simulink model "ARC_DTm"  (R2025b)
settings: Solver=FixedStepAuto  StartTime=0.0  StopTime=10080  FixedStep=1  RelTol=1e-3
PreLoadFcn:
  | %For Preload, set the working path
  | modelFolder = fileparts(which(bdroot));
  | addpath(genpath(modelFolder));
StartFcn:
  | tic
StopFcn:
  | fprintf("Sim Time: %.02f min", toc/60)
values from neighbouring files (symbols this model uses):
  batteryScenario = p.batteryScenario    [RUNSIM_ParameterSweep.m]    (also in _RUNSIM_ParameterSweep.m)
  Electricity_SalePriceModifier = 50/100    (= 0.5)    [RUNSIM_ParameterSweep.m]    (also in _RUNSIM_ParameterSweep.m)
  LUT = LUT_load.gamLUT    [RUNSIM_ParameterSweep.m]    (also in _RUNSIM_ParameterSweep.m)
  minimum_UF_system_flow = 5833    [RUNSIM_ParameterSweep.m]    (also in _RUNSIM_ParameterSweep.m)
  PROS1_recoveryrate = 61    [RUNSIM_ParameterSweep.m]    (also in _RUNSIM_ParameterSweep.m)
  PROS2_recoveryrate = 62    [RUNSIM_ParameterSweep.m]    (also in _RUNSIM_ParameterSweep.m)
  ROstabilization_time = p.ROstabilization_time    [RUNSIM_ParameterSweep.m]    (also in _RUNSIM_ParameterSweep.m)
  solarModifier = maximum_solar_generation / 300    [RUNSIM_ParameterSweep.m]    (also in _RUNSIM_ParameterSweep.m)
  TSRO_recoveryrate = 51    [RUNSIM_ParameterSweep.m]    (also in _RUNSIM_ParameterSweep.m)
  UF_RecoveryRate = 96    [RUNSIM_ParameterSweep.m]    (also in _RUNSIM_ParameterSweep.m)
undefined symbols (not defined in the file or in its folder): A_PROS1, A_PROS2, A_TSRO, B_PROS1, B_PROS2, B_TSRO, BW_Max_Time, BW_Max_Vol_gal, CEB_Max_Time, CEB_Max_Vol_gal, CIP_Max_Time, E, FF, h, L, w
libraries: simulink x40
(part 7 of 11)

== system ARC_DTm/Product Water Tank/Temperature Balance ==
  InflowLoadingRate1 : Inport
  InflowLoadingRate2 : Inport  Port=2
  OutflowRate1 (flow) : Inport  Port=3
  OutflowRate2 (FLOW) : Inport  Port=4
  Volume : Inport  Port=5
  *C*min^-1*VOL^-1 : Product  Inputs=*/
  *C/VOL : Integrator  InitialCondition=initT
  Outflow Rate (FLOW) : Sum  Inputs=|++
  Temperature Inflow Rate (*C/min) : Sum  Inputs=|++
  Temperature Outflow Rate (*C/m) : Product
  Total Loading Rate (*C/m) : Sum  Inputs=|+-
  Out1 : Outport
  wires:
  InflowLoadingRate1/1 -> Temperature Inflow Rate (*C/min)/1
  InflowLoadingRate2/1 -> Temperature Inflow Rate (*C/min)/2
  Temperature Inflow Rate (*C/min)/1 -> Total Loading Rate (*C/m)/1
  Total Loading Rate (*C/m)/1 -> *C*min^-1*VOL^-1/1
  Volume/1 -> *C*min^-1*VOL^-1/2
  *C*min^-1*VOL^-1/1 -> *C/VOL/1
  *C/VOL/1 -> Temperature Outflow Rate (*C/m)/1, Out1/1
  OutflowRate1 (flow)/1 -> Outflow Rate (FLOW)/1
  OutflowRate2 (FLOW)/1 -> Outflow Rate (FLOW)/2
  Outflow Rate (FLOW)/1 -> Temperature Outflow Rate (*C/m)/2
  Temperature Outflow Rate (*C/m)/1 -> Total Loading Rate (*C/m)/2

== system ARC_DTm/TSRO_1/Subsystem ==
  <Feed Temperature (oC)> : Inport
  <S2 Feed Pressure (bar)> : Inport  Port=2
  Pperm : Inport  Port=3
  Water Perm (L/m2/min/Bar) : Inport  Port=4
  Salt Perm (L/m2/min) : Inport  Port=5
  <S2 Feed Salinity (g/L)> : Inport  Port=6
  cperm : Inport  Port=7
  Jw : Inport  Port=8
  dh : Inport  Port=9
  L : Inport  Port=10
  u : Inport  Port=11
  MATLAB Function : MATLAB Function  TreatAsAtomicUnit=on
  Scope : Scope  NumInputPorts=3
      settings: ActiveDisplayYMinimum=-3.36183032878838E+280  ActiveDisplayYMaximum=3.0256472959095429E+281  DataLoggingVariableName=ScopeData26
  Scope1 : Scope
      settings: ActiveDisplayYMinimum=-1  ActiveDisplayYMaximum=1  DataLoggingVariableName=ScopeData28
  Permeate Flux Rate (L/min/m2) : Outport
  Permeate Salinity g/L : Outport  Port=2
  deltaPi_bar : Outport  Port=3
  wires:
  Salt Perm (L/m2/min)/1 -> MATLAB Function/5(B)
  <Feed Temperature (oC)>/1 -> MATLAB Function/1(T)
  <S2 Feed Salinity (g/L)>/1 -> Scope/1, MATLAB Function/6(cfeed)  "Feed Salinity g/L"
  <S2 Feed Pressure (bar)>/1 -> MATLAB Function/2(Pfeed)
  cperm/1 -> MATLAB Function/7(cperm_prev)
  Pperm/1 -> MATLAB Function/3(Pperm)
  Jw/1 -> MATLAB Function/8(Jw_prev)  "Permeate Flux (Jw)"
  Water Perm (L/m2/min/Bar)/1 -> MATLAB Function/4(A)
  dh/1 -> MATLAB Function/9(dh)
  L/1 -> MATLAB Function/10(L)
  u/1 -> MATLAB Function/11(u)  "Flow Velocity (cm/s)"
  MATLAB Function/1(Jw) -> Scope1/1, Permeate Flux Rate (L/min/m2)/1  "Permeate Flux Rate (L/min/m2)"
  MATLAB Function/2(cperm) -> Scope/2, Permeate Salinity g/L/1  "TSRO_1_PermeateSalinity_gL"
  MATLAB Function/3(deltaPi_bar) -> Scope/3, deltaPi_bar/1  "deltaPi_bar"

== system ARC_DTm/TSRO_2/Subsystem ==
  <Feed Temperature (oC)> : Inport
  <S2 Feed Pressure (bar)> : Inport  Port=2
  Pperm : Inport  Port=3
  Water Perm (L/m2/min/Bar) : Inport  Port=4
  Salt Perm (L/m2/min) : Inport  Port=5
  <S2 Feed Salinity (g/L)> : Inport  Port=6
  cperm : Inport  Port=7
  Jw : Inport  Port=8
  dh : Inport  Port=9
  L : Inport  Port=10
  u : Inport  Port=11
  MATLAB Function : MATLAB Function  TreatAsAtomicUnit=on
  Permeate Flux Rate (L/min/m2) : Outport
  Permeate Salinity g/L : Outport  Port=2
  deltaPi_bar : Outport  Port=3
  wires:
  Salt Perm (L/m2/min)/1 -> MATLAB Function/5(B)
  <Feed Temperature (oC)>/1 -> MATLAB Function/1(T)
  <S2 Feed Salinity (g/L)>/1 -> MATLAB Function/6(cfeed)  "Feed Salinity g/L"
  <S2 Feed Pressure (bar)>/1 -> MATLAB Function/2(Pfeed)
  cperm/1 -> MATLAB Function/7(cperm_prev)
  Pperm/1 -> MATLAB Function/3(Pperm)
  Jw/1 -> MATLAB Function/8(Jw_prev)  "Permeate Flux (Jw)"
  Water Perm (L/m2/min/Bar)/1 -> MATLAB Function/4(A)
  dh/1 -> MATLAB Function/9(dh)
  L/1 -> MATLAB Function/10(L)
  u/1 -> MATLAB Function/11(u)  "Flow Velocity (cm/s)"
  MATLAB Function/1(Jw) -> Permeate Flux Rate (L/min/m2)/1  "Permeate Flux Rate (L/min/m2)"
  MATLAB Function/2(cperm) -> Permeate Salinity g/L/1  "TSRO_2_PermeateSalinity_gL"
  MATLAB Function/3(deltaPi_bar) -> deltaPi_bar/1

== system ARC_DTm/TSRO_3/Subsystem ==
  <Feed Temperature (oC)> : Inport
  <S2 Feed Pressure (bar)> : Inport  Port=2
  Pperm : Inport  Port=3
  Water Perm (L/m2/min/Bar) : Inport  Port=4
  Salt Perm (L/m2/min) : Inport  Port=5
  <S2 Feed Salinity (g/L)> : Inport  Port=6
  cperm : Inport  Port=7
  Jw : Inport  Port=8
  dh : Inport  Port=9
  L : Inport  Port=10
  u : Inport  Port=11
  MATLAB Function : MATLAB Function  TreatAsAtomicUnit=on
  Permeate Flux Rate (L/min/m2) : Outport
  Permeate Salinity g/L : Outport  Port=2
  deltaPi_bar : Outport  Port=3
  wires:
  Salt Perm (L/m2/min)/1 -> MATLAB Function/5(B)
  <Feed Temperature (oC)>/1 -> MATLAB Function/1(T)
  <S2 Feed Salinity (g/L)>/1 -> MATLAB Function/6(cfeed)  "Feed Salinity g/L"
  <S2 Feed Pressure (bar)>/1 -> MATLAB Function/2(Pfeed)
  cperm/1 -> MATLAB Function/7(cperm_prev)
  Pperm/1 -> MATLAB Function/3(Pperm)
  Jw/1 -> MATLAB Function/8(Jw_prev)  "Permeate Flux (Jw)"
  Water Perm (L/m2/min/Bar)/1 -> MATLAB Function/4(A)
  dh/1 -> MATLAB Function/9(dh)
  L/1 -> MATLAB Function/10(L)
  u/1 -> MATLAB Function/11(u)  "Flow Velocity (cm/s)"
  MATLAB Function/1(Jw) -> Permeate Flux Rate (L/min/m2)/1  "Permeate Flux Rate (L/min/m2)"
  MATLAB Function/2(cperm) -> Permeate Salinity g/L/1  "TSRO_3_PermeateSalinity_gL"
  MATLAB Function/3(deltaPi_bar) -> deltaPi_bar/1

== system ARC_DTm/TSRO_4/Subsystem ==
  <Feed Temperature (oC)> : Inport
  <S2 Feed Pressure (bar)> : Inport  Port=2
  Pperm : Inport  Port=3
  Water Perm (L/m2/min/Bar) : Inport  Port=4
  Salt Perm (L/m2/min) : Inport  Port=5
  <S2 Feed Salinity (g/L)> : Inport  Port=6
  cperm : Inport  Port=7
  Jw : Inport  Port=8
  dh : Inport  Port=9
  L : Inport  Port=10
  u : Inport  Port=11
  MATLAB Function : MATLAB Function  TreatAsAtomicUnit=on
  Permeate Flux Rate (L/min/m2) : Outport
  Permeate Salinity g/L : Outport  Port=2
  deltaPi_bar : Outport  Port=3
  wires:
  Salt Perm (L/m2/min)/1 -> MATLAB Function/5(B)
  <Feed Temperature (oC)>/1 -> MATLAB Function/1(T)
  <S2 Feed Salinity (g/L)>/1 -> MATLAB Function/6(cfeed)  "Feed Salinity g/L"
  <S2 Feed Pressure (bar)>/1 -> MATLAB Function/2(Pfeed)
  cperm/1 -> MATLAB Function/7(cperm_prev)
  Pperm/1 -> MATLAB Function/3(Pperm)
  Jw/1 -> MATLAB Function/8(Jw_prev)  "Permeate Flux (Jw)"
  Water Perm (L/m2/min/Bar)/1 -> MATLAB Function/4(A)
  dh/1 -> MATLAB Function/9(dh)
  L/1 -> MATLAB Function/10(L)
  u/1 -> MATLAB Function/11(u)  "Flow Velocity (cm/s)"
  MATLAB Function/1(Jw) -> Permeate Flux Rate (L/min/m2)/1  "Permeate Flux Rate (L/min/m2)"
  MATLAB Function/2(cperm) -> Permeate Salinity g/L/1  "TSRO_4_PermeateSalinity_gL"
  MATLAB Function/3(deltaPi_bar) -> deltaPi_bar/1

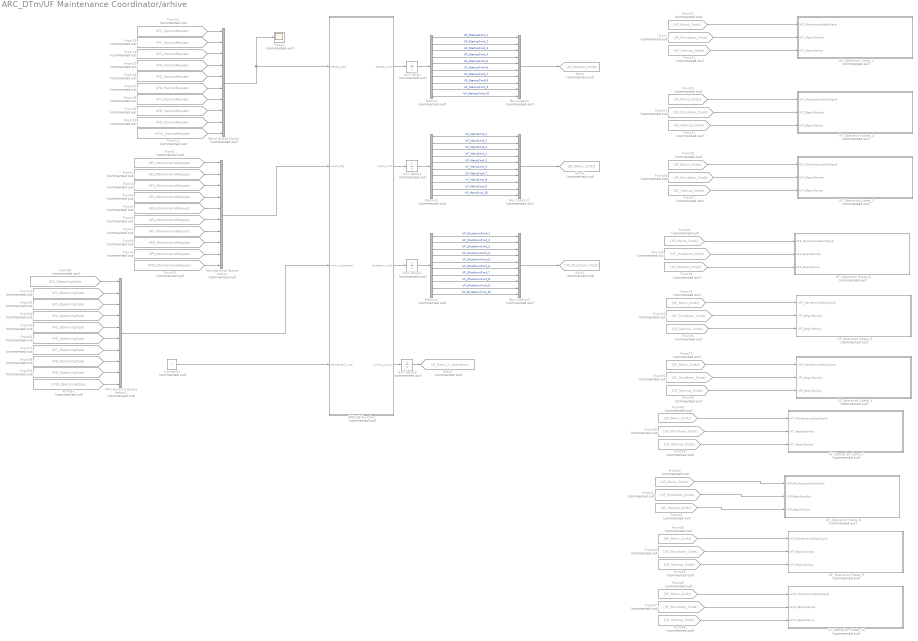
== system ARC_DTm/UF Maintenance Coordinator/arhive ==
  Bus Creator : BusCreator  Commented=on  Inputs=10
  Bus Creator1 : BusCreator  Commented=on  Inputs=10
  Bus Creator2 : BusCreator  Commented=on  Inputs=10
  Constant1 : Constant  Commented=on  Value=7
  Demux : Demux  Commented=on  Outputs=10
  Demux1 : Demux  Commented=on  Outputs=10
  Demux2 : Demux  Commented=on  Outputs=10
  From{,23,26,29,32,35,38,41,44,47} (10 alike) : From  Commented=on  GotoTag=UF_Shutdown_Cmds
  From1 : From  Commented=on  GotoTag=UF1_MaintenanceRequest  TagVisibility=global
  From10 : From  Commented=on  GotoTag=UF10_MaintenanceRequest  TagVisibility=global
  From11 : From  Commented=on  GotoTag=UF1_StartupRequest  TagVisibility=global
  From12 : From  Commented=on  GotoTag=UF10_StartupRequest  TagVisibility=global
  From13 : From  Commented=on  GotoTag=UF2_StartupRequest  TagVisibility=global
  From14 : From  Commented=on  GotoTag=UF3_StartupRequest  TagVisibility=global
  From15 : From  Commented=on  GotoTag=UF4_StartupRequest  TagVisibility=global
  From16 : From  Commented=on  GotoTag=UF5_StartupRequest  TagVisibility=global
  From17 : From  Commented=on  GotoTag=UF6_StartupRequest  TagVisibility=global
  From18 : From  Commented=on  GotoTag=UF7_StartupRequest  TagVisibility=global
  From19 : From  Commented=on  GotoTag=UF8_StartupRequest  TagVisibility=global
  From2 : From  Commented=on  GotoTag=UF2_MaintenanceRequest  TagVisibility=global
  From20 : From  Commented=on  GotoTag=UF9_StartupRequest  TagVisibility=global
  From{21,24,27,30,33,36,39,42,45,48} (10 alike) : From  Commented=on  GotoTag=UF_Startup_Cmds
  From{22,25,28,31,34,37,40,43,46,49} (10 alike) : From  Commented=on  GotoTag=UF_Maint_Cmds
  From3 : From  Commented=on  GotoTag=UF3_MaintenanceRequest  TagVisibility=global
  From4 : From  Commented=on  GotoTag=UF4_MaintenanceRequest  TagVisibility=global
  From5 : From  Commented=on  GotoTag=UF5_MaintenanceRequest  TagVisibility=global
  From50 : From  Commented=on  GotoTag=UF1_OperatingState  TagVisibility=global
  From51 : From  Commented=on  GotoTag=UF10_OperatingState  TagVisibility=global
  From52 : From  Commented=on  GotoTag=UF2_OperatingState  TagVisibility=global
  From53 : From  Commented=on  GotoTag=UF3_OperatingState  TagVisibility=global
  From54 : From  Commented=on  GotoTag=UF4_OperatingState  TagVisibility=global
  From55 : From  Commented=on  GotoTag=UF5_OperatingState  TagVisibility=global
  From56 : From  Commented=on  GotoTag=UF6_OperatingState  TagVisibility=global
  From57 : From  Commented=on  GotoTag=UF7_OperatingState  TagVisibility=global
  From58 : From  Commented=on  GotoTag=UF8_OperatingState  TagVisibility=global
  From59 : From  Commented=on  GotoTag=UF9_OperatingState  TagVisibility=global
  From6 : From  Commented=on  GotoTag=UF6_MaintenanceRequest  TagVisibility=global
  From7 : From  Commented=on  GotoTag=UF7_MaintenanceRequest  TagVisibility=global
  From8 : From  Commented=on  GotoTag=UF8_MaintenanceRequest  TagVisibility=global
  From9 : From  Commented=on  GotoTag=UF9_MaintenanceRequest  TagVisibility=global
  Goto : Goto  Commented=on  GotoTag=UF_Startup_Cmds
  Goto1 : Goto  Commented=on  GotoTag=UF_Maint_Cmds
  Goto2 : Goto  Commented=on  GotoTag=UF_Shutdown_Cmds
  Goto3 : Goto  Commented=on  GotoTag=UF_Units_in_operations  TagVisibility=global
  MATLAB Function : MATLAB Function  Priority=100  Commented=on  TreatAsAtomicUnit=on
  Maint Queue Vector : Mux  Commented=on  Inputs=10
  Maintenance Queue Vector : Mux  Commented=on  Inputs=10
  Maintenance Queue Vector1 : Mux  Commented=on  Inputs=10
  Scope : Scope  Commented=on
      settings: ActiveDisplayYMinimum=0.31827009128781919  ActiveDisplayYMaximum=0.91954146390153213
  UF_Operation State_1 : Subsystem  Commented=on
  UF_Operation State_10 : Subsystem  Commented=on
  UF_Operation State_2 : Subsystem  Commented=on
  UF_Operation State_3 : Subsystem  Commented=on
  UF_Operation State_4 : Subsystem  Commented=on
  UF_Operation State_5 : Subsystem  Commented=on
  UF_Operation State_6 : Subsystem  Commented=on
  UF_Operation State_7 : Subsystem  Commented=on
  UF_Operation State_8 : Subsystem  Commented=on
  UF_Operation State_9 : Subsystem  Commented=on
  Unit Delay{,1..3} (4 alike) : UnitDelay  Commented=on  SampleTime=-1  HasFrameUpgradeWarning=on
  wires:
  Demux2/9 -> Bus Creator2/9  "UF_ShutdownCmd_9"
  From13/1 -> Maint Queue Vector/2
  From42/1 -> UF_Operation State_8/3(UF8_BeginStartup)
  From48/1 -> UF_Operation State_10/3(UF10_BeginStartup)
  Demux2/10 -> Bus Creator2/10  "UF_ShutdownCmd_10"
  From47/1 -> UF_Operation State_10/2(UF10_BeginStandby)
  Demux2/6 -> Bus Creator2/6  "UF_ShutdownCmd_6"
  Demux1/6 -> Bus Creator1/6  "UF_MaintCmd_6"
  From24/1 -> UF_Operation State_2/3(UF2_BeginStartup)
  Maintenance Queue Vector/1 -> MATLAB Function/2(maint_req)
  From1/1 -> Maintenance Queue Vector/1
  From23/1 -> UF_Operation State_2/2(UF2_BeginStandby)
  MATLAB Function/3(shutdown_cmd) -> Unit Delay2/1
  From30/1 -> UF_Operation State_4/3(UF4_BeginStartup)
  From57/1 -> Maintenance Queue Vector1/7
  Unit Delay/1 -> Demux/1
  Demux/10 -> Bus Creator/10  "UF_StartupCmd_10"
  From54/1 -> Maintenance Queue Vector1/4
  From45/1 -> UF_Operation State_9/3(UF9_BeginStartup)
  Demux1/2 -> Bus Creator1/2  "UF_MaintCmd_2"
  From7/1 -> Maintenance Queue Vector/7
  From58/1 -> Maintenance Queue Vector1/8
  From49/1 -> UF_Operation State_10/1(UF10_MaintenanceStartSignal)
  From29/1 -> UF_Operation State_4/2(UF4_BeginStandby)
  From6/1 -> Maintenance Queue Vector/6
  From10/1 -> Maintenance Queue Vector/10
  From56/1 -> Maintenance Queue Vector1/6
  From33/1 -> UF_Operation State_5/3(UF5_BeginStartup)
  From31/1 -> UF_Operation State_4/1(UF4_MaintenanceStartSignal)
  From/1 -> UF_Operation State_1/2(UF1_BeginStandby)
  From53/1 -> Maintenance Queue Vector1/3
  From34/1 -> UF_Operation State_5/1(UF5_MaintenanceStartSignal)
  Demux2/5 -> Bus Creator2/5  "UF_ShutdownCmd_5"
  Unit Delay3/1 -> Goto3/1
  From59/1 -> Maintenance Queue Vector1/9
  Demux/7 -> Bus Creator/7  "UF_StartupCmd_7"
  Maintenance Queue Vector1/1 -> MATLAB Function/3(unit_in_operation)
  Demux2/7 -> Bus Creator2/7  "UF_ShutdownCmd_7"
  From3/1 -> Maintenance Queue Vector/3
  From38/1 -> UF_Operation State_7/2(UF7_BeginStandby)
  From40/1 -> UF_Operation State_7/1(UF7_MaintenanceStartSignal)
  From26/1 -> UF_Operation State_3/2(UF3_BeginStandby)
  Bus Creator1/1 -> Goto1/1
  From2/1 -> Maintenance Queue Vector/2
  Demux2/3 -> Bus Creator2/3  "UF_ShutdownCmd_3"
  From39/1 -> UF_Operation State_7/3(UF7_BeginStartup)
  Demux1/9 -> Bus Creator1/9  "UF_MaintCmd_9"
  Demux2/2 -> Bus Creator2/2  "UF_ShutdownCmd_2"
  From46/1 -> UF_Operation State_9/1(UF9_MaintenanceStartSignal)
  From20/1 -> Maint Queue Vector/9
  Demux/4 -> Bus Creator/4  "UF_StartupCmd_4"
  Demux2/4 -> Bus Creator2/4  "UF_ShutdownCmd_4"
  Demux/5 -> Bus Creator/5  "UF_StartupCmd_5"
  Demux2/1 -> Bus Creator2/1  "UF_ShutdownCmd_1"
  From9/1 -> Maintenance Queue Vector/9
  From32/1 -> UF_Operation State_5/2(UF5_BeginStandby)
  Demux1/3 -> Bus Creator1/3  "UF_MaintCmd_3"
  Demux1/5 -> Bus Creator1/5  "UF_MaintCmd_5"
  From55/1 -> Maintenance Queue Vector1/5
  From4/1 -> Maintenance Queue Vector/4
  MATLAB Function/4(running_count) -> Unit Delay3/1
  Demux/6 -> Bus Creator/6  "UF_StartupCmd_6"
  From22/1 -> UF_Operation State_1/1(UF1_MaintenanceStartSignal)
  Demux/8 -> Bus Creator/8  "UF_StartupCmd_8"
  Demux/9 -> Bus Creator/9  "UF_StartupCmd_9"
  From8/1 -> Maintenance Queue Vector/8
  Demux1/1 -> Bus Creator1/1  "UF_MaintCmd_1"
  Demux1/10 -> Bus Creator1/10  "UF_MaintCmd_10"
  From50/1 -> Maintenance Queue Vector1/1
  Demux1/4 -> Bus Creator1/4  "UF_MaintCmd_4"
  MATLAB Function/1(startup_cmd) -> Unit Delay/1
  From52/1 -> Maintenance Queue Vector1/2
  From27/1 -> UF_Operation State_3/3(UF3_BeginStartup)
  From15/1 -> Maint Queue Vector/4
  From51/1 -> Maintenance Queue Vector1/10
  From36/1 -> UF_Operation State_6/3(UF6_BeginStartup)
  MATLAB Function/2(maint_cmd) -> Unit Delay1/1
  Unit Delay2/1 -> Demux2/1
  From43/1 -> UF_Operation State_8/1(UF8_MaintenanceStartSignal)
  From28/1 -> UF_Operation State_3/1(UF3_MaintenanceStartSignal)
  Demux2/8 -> Bus Creator2/8  "UF_ShutdownCmd_8"
  Demux/2 -> Bus Creator/2  "UF_StartupCmd_2"
  From35/1 -> UF_Operation State_6/2(UF6_BeginStandby)
  Bus Creator2/1 -> Goto2/1
  Bus Creator/1 -> Goto/1
  From37/1 -> UF_Operation State_6/1(UF6_MaintenanceStartSignal)
  Constant1/1 -> MATLAB Function/4(demanded_units)
  Demux1/8 -> Bus Creator1/8  "UF_MaintCmd_8"
  From25/1 -> UF_Operation State_2/1(UF2_MaintenanceStartSignal)
  From44/1 -> UF_Operation State_9/2(UF9_BeginStandby)
  Demux1/7 -> Bus Creator1/7  "UF_MaintCmd_7"
  Demux/3 -> Bus Creator/3  "UF_StartupCmd_3"
  Demux/1 -> Bus Creator/1  "UF_StartupCmd_1"
  From41/1 -> UF_Operation State_8/2(UF8_BeginStandby)
  From21/1 -> UF_Operation State_1/3(UF1_BeginStartup)
  From5/1 -> Maintenance Queue Vector/5
  Unit Delay1/1 -> Demux1/1
  From16/1 -> Maint Queue Vector/5
  From17/1 -> Maint Queue Vector/6
  From19/1 -> Maint Queue Vector/8
  From11/1 -> Maint Queue Vector/1
  From12/1 -> Maint Queue Vector/10
  From18/1 -> Maint Queue Vector/7
  Maint Queue Vector/1 -> Scope/1, MATLAB Function/1(startup_req)
  From14/1 -> Maint Queue Vector/3

== system ARC_DTm/UF1/Subsystem ==
  note: The GAM utilizes smoothing functions to generate non-interacting linear regressions between the parameters. The format of the equation is as such:
      | $y = \beta_0 + \sum_{n=1}^N{f_n(x_n)}\\ f_n(x_n) = \beta_{n}*sm_n(x_n)$
      | where f_n is the weighted smoothing function for variable n across the set N. Each 1-D lookup table below represents the weighted smooth function output for the respective variable. This GAM lookup table approach provided a more computationally efficient method to predict using the GAM at very minor losses in fidelity ( ~0.1% MAPE from raw GAM outputs across a test set).
  t_BW : Inport
  t_CEB : Inport  Port=2
  t_CIP : Inport  Port=3
  V_BW : Inport  Port=4
  V_CEB : Inport  Port=5
  Feed Turbidity : Inport  Port=6
  T : Inport  Port=7
  B1: t_BW : Lookup_n-D  NumberOfTableDimensions=1  BreakpointsForDimension1=LUT.breakpoints(:,3)  Table=LUT.values(:,3)  ExtrapMethod=Clip  InternalRulePriority=Speed  RndMeth=Simplest
  B2: t_CEB : Lookup_n-D  NumberOfTableDimensions=1  BreakpointsForDimension1=LUT.breakpoints(:,5)  Table=LUT.values(:,5)  ExtrapMethod=Clip  InternalRulePriority=Speed  RndMeth=Simplest
  B3: t_CIP : Lookup_n-D  NumberOfTableDimensions=1  BreakpointsForDimension1=LUT.breakpoints(:,4)  Table=LUT.values(:,4)  ExtrapMethod=Clip  InternalRulePriority=Speed  RndMeth=Simplest
  B4: V_BW : Lookup_n-D  NumberOfTableDimensions=1  BreakpointsForDimension1=LUT.breakpoints(:,6)  Table=LUT.values(:,6)  ExtrapMethod=Clip  InternalRulePriority=Speed  RndMeth=Simplest
  B5: V_CEB : Lookup_n-D  NumberOfTableDimensions=1  BreakpointsForDimension1=LUT.breakpoints(:,7)  Table=LUT.values(:,7)  ExtrapMethod=Clip  InternalRulePriority=Speed  RndMeth=Simplest
  B6: Turbidity : Lookup_n-D  NumberOfTableDimensions=1  BreakpointsForDimension1=LUT.breakpoints(:,1)  Table=LUT.values(:,1)  ExtrapMethod=Clip  InternalRulePriority=Speed  RndMeth=Simplest
  B7: Temperature : Lookup_n-D  NumberOfTableDimensions=1  BreakpointsForDimension1=LUT.breakpoints(:,2)  Table=LUT.values(:,2)  ExtrapMethod=Clip  InternalRulePriority=Speed  RndMeth=Simplest
  Intercept : Constant  Value=LUT.intercept
  Sum : Sum  Inputs=++++++++
  A_UF : Outport
  wires:
  Sum/1 -> A_UF/1
  t_BW/1 -> B1: t_BW/1
  B1: t_BW/1 -> Sum/2
  Intercept/1 -> Sum/1
  t_CEB/1 -> B2: t_CEB/1
  B2: t_CEB/1 -> Sum/3
  t_CIP/1 -> B3: t_CIP/1
  B3: t_CIP/1 -> Sum/4
  V_BW/1 -> B4: V_BW/1
  B4: V_BW/1 -> Sum/5
  V_CEB/1 -> B5: V_CEB/1
  B5: V_CEB/1 -> Sum/6
  B6: Turbidity/1 -> Sum/7
  Feed Turbidity/1 -> B6: Turbidity/1
  T/1 -> B7: Temperature/1
  B7: Temperature/1 -> Sum/8

== system ARC_DTm/UF10/Subsystem ==
  note: The GAM utilizes smoothing functions to generate non-interacting linear regressions between the parameters. The format of the equation is as such:
      | $y = \beta_0 + \sum_{n=1}^N{f_n(x_n)}\\ f_n(x_n) = \beta_{n}*sm_n(x_n)$
      | where f_n is the weighted smoothing function for variable n across the set N. Each 1-D lookup table below represents the weighted smooth function output for the respective variable. This GAM lookup table approach provided a more computationally efficient method to predict using the GAM at very minor losses in fidelity ( ~0.1% MAPE from raw GAM outputs across a test set).
  t_BW : Inport
  t_CEB : Inport  Port=2
  t_CIP : Inport  Port=3
  V_BW : Inport  Port=4
  V_CEB : Inport  Port=5
  Feed Turbidity : Inport  Port=6
  T : Inport  Port=7
  B1: t_BW : Lookup_n-D  NumberOfTableDimensions=1  BreakpointsForDimension1=LUT.breakpoints(:,3)  Table=LUT.values(:,3)  ExtrapMethod=Clip  InternalRulePriority=Speed  RndMeth=Simplest
  B2: t_CEB : Lookup_n-D  NumberOfTableDimensions=1  BreakpointsForDimension1=LUT.breakpoints(:,5)  Table=LUT.values(:,5)  ExtrapMethod=Clip  InternalRulePriority=Speed  RndMeth=Simplest
  B3: t_CIP : Lookup_n-D  NumberOfTableDimensions=1  BreakpointsForDimension1=LUT.breakpoints(:,4)  Table=LUT.values(:,4)  ExtrapMethod=Clip  InternalRulePriority=Speed  RndMeth=Simplest
  B4: V_BW : Lookup_n-D  NumberOfTableDimensions=1  BreakpointsForDimension1=LUT.breakpoints(:,6)  Table=LUT.values(:,6)  ExtrapMethod=Clip  InternalRulePriority=Speed  RndMeth=Simplest
  B5: V_CEB : Lookup_n-D  NumberOfTableDimensions=1  BreakpointsForDimension1=LUT.breakpoints(:,7)  Table=LUT.values(:,7)  ExtrapMethod=Clip  InternalRulePriority=Speed  RndMeth=Simplest
  B6: Turbidity : Lookup_n-D  NumberOfTableDimensions=1  BreakpointsForDimension1=LUT.breakpoints(:,1)  Table=LUT.values(:,1)  ExtrapMethod=Clip  InternalRulePriority=Speed  RndMeth=Simplest
  B7: Temperature : Lookup_n-D  NumberOfTableDimensions=1  BreakpointsForDimension1=LUT.breakpoints(:,2)  Table=LUT.values(:,2)  ExtrapMethod=Clip  InternalRulePriority=Speed  RndMeth=Simplest
  Intercept : Constant  Value=LUT.intercept
  Sum : Sum  Inputs=++++++++
  A_UF : Outport
  wires:
  Sum/1 -> A_UF/1
  t_BW/1 -> B1: t_BW/1
  B1: t_BW/1 -> Sum/2
  Intercept/1 -> Sum/1
  t_CEB/1 -> B2: t_CEB/1
  B2: t_CEB/1 -> Sum/3
  t_CIP/1 -> B3: t_CIP/1
  B3: t_CIP/1 -> Sum/4
  V_BW/1 -> B4: V_BW/1
  B4: V_BW/1 -> Sum/5
  V_CEB/1 -> B5: V_CEB/1
  B5: V_CEB/1 -> Sum/6
  B6: Turbidity/1 -> Sum/7
  Feed Turbidity/1 -> B6: Turbidity/1
  T/1 -> B7: Temperature/1
  B7: Temperature/1 -> Sum/8

== system ARC_DTm/UF2/Subsystem ==
  note: The GAM utilizes smoothing functions to generate non-interacting linear regressions between the parameters. The format of the equation is as such:
      | $y = \beta_0 + \sum_{n=1}^N{f_n(x_n)}\\ f_n(x_n) = \beta_{n}*sm_n(x_n)$
      | where f_n is the weighted smoothing function for variable n across the set N. Each 1-D lookup table below represents the weighted smooth function output for the respective variable. This GAM lookup table approach provided a more computationally efficient method to predict using the GAM at very minor losses in fidelity ( ~0.1% MAPE from raw GAM outputs across a test set).
  t_BW : Inport
  t_CEB : Inport  Port=2
  t_CIP : Inport  Port=3
  V_BW : Inport  Port=4
  V_CEB : Inport  Port=5
  Feed Turbidity : Inport  Port=6
  T : Inport  Port=7
  B1: t_BW : Lookup_n-D  NumberOfTableDimensions=1  BreakpointsForDimension1=LUT.breakpoints(:,3)  Table=LUT.values(:,3)  ExtrapMethod=Clip  InternalRulePriority=Speed  RndMeth=Simplest
  B2: t_CEB : Lookup_n-D  NumberOfTableDimensions=1  BreakpointsForDimension1=LUT.breakpoints(:,5)  Table=LUT.values(:,5)  ExtrapMethod=Clip  InternalRulePriority=Speed  RndMeth=Simplest
  B3: t_CIP : Lookup_n-D  NumberOfTableDimensions=1  BreakpointsForDimension1=LUT.breakpoints(:,4)  Table=LUT.values(:,4)  ExtrapMethod=Clip  InternalRulePriority=Speed  RndMeth=Simplest
  B4: V_BW : Lookup_n-D  NumberOfTableDimensions=1  BreakpointsForDimension1=LUT.breakpoints(:,6)  Table=LUT.values(:,6)  ExtrapMethod=Clip  InternalRulePriority=Speed  RndMeth=Simplest
  B5: V_CEB : Lookup_n-D  NumberOfTableDimensions=1  BreakpointsForDimension1=LUT.breakpoints(:,7)  Table=LUT.values(:,7)  ExtrapMethod=Clip  InternalRulePriority=Speed  RndMeth=Simplest
  B6: Turbidity : Lookup_n-D  NumberOfTableDimensions=1  BreakpointsForDimension1=LUT.breakpoints(:,1)  Table=LUT.values(:,1)  ExtrapMethod=Clip  InternalRulePriority=Speed  RndMeth=Simplest
  B7: Temperature : Lookup_n-D  NumberOfTableDimensions=1  BreakpointsForDimension1=LUT.breakpoints(:,2)  Table=LUT.values(:,2)  ExtrapMethod=Clip  InternalRulePriority=Speed  RndMeth=Simplest
  Intercept : Constant  Value=LUT.intercept
  Sum : Sum  Inputs=++++++++
  A_UF : Outport
  wires:
  Sum/1 -> A_UF/1
  t_BW/1 -> B1: t_BW/1
  B1: t_BW/1 -> Sum/2
  Intercept/1 -> Sum/1
  t_CEB/1 -> B2: t_CEB/1
  B2: t_CEB/1 -> Sum/3
  t_CIP/1 -> B3: t_CIP/1
  B3: t_CIP/1 -> Sum/4
  V_BW/1 -> B4: V_BW/1
  B4: V_BW/1 -> Sum/5
  V_CEB/1 -> B5: V_CEB/1
  B5: V_CEB/1 -> Sum/6
  B6: Turbidity/1 -> Sum/7
  Feed Turbidity/1 -> B6: Turbidity/1
  T/1 -> B7: Temperature/1
  B7: Temperature/1 -> Sum/8

== system ARC_DTm/UF3/Subsystem ==
  note: The GAM utilizes smoothing functions to generate non-interacting linear regressions between the parameters. The format of the equation is as such:
      | $y = \beta_0 + \sum_{n=1}^N{f_n(x_n)}\\ f_n(x_n) = \beta_{n}*sm_n(x_n)$
      | where f_n is the weighted smoothing function for variable n across the set N. Each 1-D lookup table below represents the weighted smooth function output for the respective variable. This GAM lookup table approach provided a more computationally efficient method to predict using the GAM at very minor losses in fidelity ( ~0.1% MAPE from raw GAM outputs across a test set).
  t_BW : Inport
  t_CEB : Inport  Port=2
  t_CIP : Inport  Port=3
  V_BW : Inport  Port=4
  V_CEB : Inport  Port=5
  Feed Turbidity : Inport  Port=6
  T : Inport  Port=7
  B1: t_BW : Lookup_n-D  NumberOfTableDimensions=1  BreakpointsForDimension1=LUT.breakpoints(:,3)  Table=LUT.values(:,3)  ExtrapMethod=Clip  InternalRulePriority=Speed  RndMeth=Simplest
  B2: t_CEB : Lookup_n-D  NumberOfTableDimensions=1  BreakpointsForDimension1=LUT.breakpoints(:,5)  Table=LUT.values(:,5)  ExtrapMethod=Clip  InternalRulePriority=Speed  RndMeth=Simplest
  B3: t_CIP : Lookup_n-D  NumberOfTableDimensions=1  BreakpointsForDimension1=LUT.breakpoints(:,4)  Table=LUT.values(:,4)  ExtrapMethod=Clip  InternalRulePriority=Speed  RndMeth=Simplest
  B4: V_BW : Lookup_n-D  NumberOfTableDimensions=1  BreakpointsForDimension1=LUT.breakpoints(:,6)  Table=LUT.values(:,6)  ExtrapMethod=Clip  InternalRulePriority=Speed  RndMeth=Simplest
  B5: V_CEB : Lookup_n-D  NumberOfTableDimensions=1  BreakpointsForDimension1=LUT.breakpoints(:,7)  Table=LUT.values(:,7)  ExtrapMethod=Clip  InternalRulePriority=Speed  RndMeth=Simplest
  B6: Turbidity : Lookup_n-D  NumberOfTableDimensions=1  BreakpointsForDimension1=LUT.breakpoints(:,1)  Table=LUT.values(:,1)  ExtrapMethod=Clip  InternalRulePriority=Speed  RndMeth=Simplest
  B7: Temperature : Lookup_n-D  NumberOfTableDimensions=1  BreakpointsForDimension1=LUT.breakpoints(:,2)  Table=LUT.values(:,2)  ExtrapMethod=Clip  InternalRulePriority=Speed  RndMeth=Simplest
  Intercept : Constant  Value=LUT.intercept
  Sum : Sum  Inputs=++++++++
  A_UF : Outport
  wires:
  Sum/1 -> A_UF/1
  t_BW/1 -> B1: t_BW/1
  B1: t_BW/1 -> Sum/2
  Intercept/1 -> Sum/1
  t_CEB/1 -> B2: t_CEB/1
  B2: t_CEB/1 -> Sum/3
  t_CIP/1 -> B3: t_CIP/1
  B3: t_CIP/1 -> Sum/4
  V_BW/1 -> B4: V_BW/1
  B4: V_BW/1 -> Sum/5
  V_CEB/1 -> B5: V_CEB/1
  B5: V_CEB/1 -> Sum/6
  B6: Turbidity/1 -> Sum/7
  Feed Turbidity/1 -> B6: Turbidity/1
  T/1 -> B7: Temperature/1
  B7: Temperature/1 -> Sum/8

== system ARC_DTm/UF4/Subsystem ==
  note: The GAM utilizes smoothing functions to generate non-interacting linear regressions between the parameters. The format of the equation is as such:
      | $y = \beta_0 + \sum_{n=1}^N{f_n(x_n)}\\ f_n(x_n) = \beta_{n}*sm_n(x_n)$
      | where f_n is the weighted smoothing function for variable n across the set N. Each 1-D lookup table below represents the weighted smooth function output for the respective variable. This GAM lookup table approach provided a more computationally efficient method to predict using the GAM at very minor losses in fidelity ( ~0.1% MAPE from raw GAM outputs across a test set).
  t_BW : Inport
  t_CEB : Inport  Port=2
  t_CIP : Inport  Port=3
  V_BW : Inport  Port=4
  V_CEB : Inport  Port=5
  Feed Turbidity : Inport  Port=6
  T : Inport  Port=7
  B1: t_BW : Lookup_n-D  NumberOfTableDimensions=1  BreakpointsForDimension1=LUT.breakpoints(:,3)  Table=LUT.values(:,3)  ExtrapMethod=Clip  InternalRulePriority=Speed  RndMeth=Simplest
  B2: t_CEB : Lookup_n-D  NumberOfTableDimensions=1  BreakpointsForDimension1=LUT.breakpoints(:,5)  Table=LUT.values(:,5)  ExtrapMethod=Clip  InternalRulePriority=Speed  RndMeth=Simplest
  B3: t_CIP : Lookup_n-D  NumberOfTableDimensions=1  BreakpointsForDimension1=LUT.breakpoints(:,4)  Table=LUT.values(:,4)  ExtrapMethod=Clip  InternalRulePriority=Speed  RndMeth=Simplest
  B4: V_BW : Lookup_n-D  NumberOfTableDimensions=1  BreakpointsForDimension1=LUT.breakpoints(:,6)  Table=LUT.values(:,6)  ExtrapMethod=Clip  InternalRulePriority=Speed  RndMeth=Simplest
  B5: V_CEB : Lookup_n-D  NumberOfTableDimensions=1  BreakpointsForDimension1=LUT.breakpoints(:,7)  Table=LUT.values(:,7)  ExtrapMethod=Clip  InternalRulePriority=Speed  RndMeth=Simplest
  B6: Turbidity : Lookup_n-D  NumberOfTableDimensions=1  BreakpointsForDimension1=LUT.breakpoints(:,1)  Table=LUT.values(:,1)  ExtrapMethod=Clip  InternalRulePriority=Speed  RndMeth=Simplest
  B7: Temperature : Lookup_n-D  NumberOfTableDimensions=1  BreakpointsForDimension1=LUT.breakpoints(:,2)  Table=LUT.values(:,2)  ExtrapMethod=Clip  InternalRulePriority=Speed  RndMeth=Simplest
  Intercept : Constant  Value=LUT.intercept
  Sum : Sum  Inputs=++++++++
  A_UF : Outport
  wires:
  Sum/1 -> A_UF/1
  t_BW/1 -> B1: t_BW/1
  B1: t_BW/1 -> Sum/2
  Intercept/1 -> Sum/1
  t_CEB/1 -> B2: t_CEB/1
  B2: t_CEB/1 -> Sum/3
  t_CIP/1 -> B3: t_CIP/1
  B3: t_CIP/1 -> Sum/4
  V_BW/1 -> B4: V_BW/1
  B4: V_BW/1 -> Sum/5
  V_CEB/1 -> B5: V_CEB/1
  B5: V_CEB/1 -> Sum/6
  B6: Turbidity/1 -> Sum/7
  Feed Turbidity/1 -> B6: Turbidity/1
  T/1 -> B7: Temperature/1
  B7: Temperature/1 -> Sum/8

== system ARC_DTm/UF5/Subsystem ==
  note: The GAM utilizes smoothing functions to generate non-interacting linear regressions between the parameters. The format of the equation is as such:
      | $y = \beta_0 + \sum_{n=1}^N{f_n(x_n)}\\ f_n(x_n) = \beta_{n}*sm_n(x_n)$
      | where f_n is the weighted smoothing function for variable n across the set N. Each 1-D lookup table below represents the weighted smooth function output for the respective variable. This GAM lookup table approach provided a more computationally efficient method to predict using the GAM at very minor losses in fidelity ( ~0.1% MAPE from raw GAM outputs across a test set).
  t_BW : Inport
  t_CEB : Inport  Port=2
  t_CIP : Inport  Port=3
  V_BW : Inport  Port=4
  V_CEB : Inport  Port=5
  Feed Turbidity : Inport  Port=6
  T : Inport  Port=7
  B1: t_BW : Lookup_n-D  NumberOfTableDimensions=1  BreakpointsForDimension1=LUT.breakpoints(:,3)  Table=LUT.values(:,3)  ExtrapMethod=Clip  InternalRulePriority=Speed  RndMeth=Simplest
  B2: t_CEB : Lookup_n-D  NumberOfTableDimensions=1  BreakpointsForDimension1=LUT.breakpoints(:,5)  Table=LUT.values(:,5)  ExtrapMethod=Clip  InternalRulePriority=Speed  RndMeth=Simplest
  B3: t_CIP : Lookup_n-D  NumberOfTableDimensions=1  BreakpointsForDimension1=LUT.breakpoints(:,4)  Table=LUT.values(:,4)  ExtrapMethod=Clip  InternalRulePriority=Speed  RndMeth=Simplest
  B4: V_BW : Lookup_n-D  NumberOfTableDimensions=1  BreakpointsForDimension1=LUT.breakpoints(:,6)  Table=LUT.values(:,6)  ExtrapMethod=Clip  InternalRulePriority=Speed  RndMeth=Simplest
  B5: V_CEB : Lookup_n-D  NumberOfTableDimensions=1  BreakpointsForDimension1=LUT.breakpoints(:,7)  Table=LUT.values(:,7)  ExtrapMethod=Clip  InternalRulePriority=Speed  RndMeth=Simplest
  B6: Turbidity : Lookup_n-D  NumberOfTableDimensions=1  BreakpointsForDimension1=LUT.breakpoints(:,1)  Table=LUT.values(:,1)  ExtrapMethod=Clip  InternalRulePriority=Speed  RndMeth=Simplest
  B7: Temperature : Lookup_n-D  NumberOfTableDimensions=1  BreakpointsForDimension1=LUT.breakpoints(:,2)  Table=LUT.values(:,2)  ExtrapMethod=Clip  InternalRulePriority=Speed  RndMeth=Simplest
  Intercept : Constant  Value=LUT.intercept
  Sum : Sum  Inputs=++++++++
  A_UF : Outport
  wires:
  Sum/1 -> A_UF/1
  t_BW/1 -> B1: t_BW/1
  B1: t_BW/1 -> Sum/2
  Intercept/1 -> Sum/1
  t_CEB/1 -> B2: t_CEB/1
  B2: t_CEB/1 -> Sum/3
  t_CIP/1 -> B3: t_CIP/1
  B3: t_CIP/1 -> Sum/4
  V_BW/1 -> B4: V_BW/1
  B4: V_BW/1 -> Sum/5
  V_CEB/1 -> B5: V_CEB/1
  B5: V_CEB/1 -> Sum/6
  B6: Turbidity/1 -> Sum/7
  Feed Turbidity/1 -> B6: Turbidity/1
  T/1 -> B7: Temperature/1
  B7: Temperature/1 -> Sum/8

== system ARC_DTm/UF6/Subsystem ==
  note: The GAM utilizes smoothing functions to generate non-interacting linear regressions between the parameters. The format of the equation is as such:
      | $y = \beta_0 + \sum_{n=1}^N{f_n(x_n)}\\ f_n(x_n) = \beta_{n}*sm_n(x_n)$
      | where f_n is the weighted smoothing function for variable n across the set N. Each 1-D lookup table below represents the weighted smooth function output for the respective variable. This GAM lookup table approach provided a more computationally efficient method to predict using the GAM at very minor losses in fidelity ( ~0.1% MAPE from raw GAM outputs across a test set).
  t_BW : Inport
  t_CEB : Inport  Port=2
  t_CIP : Inport  Port=3
  V_BW : Inport  Port=4
  V_CEB : Inport  Port=5
  Feed Turbidity : Inport  Port=6
  T : Inport  Port=7
  B1: t_BW : Lookup_n-D  NumberOfTableDimensions=1  BreakpointsForDimension1=LUT.breakpoints(:,3)  Table=LUT.values(:,3)  ExtrapMethod=Clip  InternalRulePriority=Speed  RndMeth=Simplest
  B2: t_CEB : Lookup_n-D  NumberOfTableDimensions=1  BreakpointsForDimension1=LUT.breakpoints(:,5)  Table=LUT.values(:,5)  ExtrapMethod=Clip  InternalRulePriority=Speed  RndMeth=Simplest
  B3: t_CIP : Lookup_n-D  NumberOfTableDimensions=1  BreakpointsForDimension1=LUT.breakpoints(:,4)  Table=LUT.values(:,4)  ExtrapMethod=Clip  InternalRulePriority=Speed  RndMeth=Simplest
  B4: V_BW : Lookup_n-D  NumberOfTableDimensions=1  BreakpointsForDimension1=LUT.breakpoints(:,6)  Table=LUT.values(:,6)  ExtrapMethod=Clip  InternalRulePriority=Speed  RndMeth=Simplest
  B5: V_CEB : Lookup_n-D  NumberOfTableDimensions=1  BreakpointsForDimension1=LUT.breakpoints(:,7)  Table=LUT.values(:,7)  ExtrapMethod=Clip  InternalRulePriority=Speed  RndMeth=Simplest
  B6: Turbidity : Lookup_n-D  NumberOfTableDimensions=1  BreakpointsForDimension1=LUT.breakpoints(:,1)  Table=LUT.values(:,1)  ExtrapMethod=Clip  InternalRulePriority=Speed  RndMeth=Simplest
  B7: Temperature : Lookup_n-D  NumberOfTableDimensions=1  BreakpointsForDimension1=LUT.breakpoints(:,2)  Table=LUT.values(:,2)  ExtrapMethod=Clip  InternalRulePriority=Speed  RndMeth=Simplest
  Intercept : Constant  Value=LUT.intercept
  Sum : Sum  Inputs=++++++++
  A_UF : Outport
  wires:
  Sum/1 -> A_UF/1
  t_BW/1 -> B1: t_BW/1
  B1: t_BW/1 -> Sum/2
  Intercept/1 -> Sum/1
  t_CEB/1 -> B2: t_CEB/1
  B2: t_CEB/1 -> Sum/3
  t_CIP/1 -> B3: t_CIP/1
  B3: t_CIP/1 -> Sum/4
  V_BW/1 -> B4: V_BW/1
  B4: V_BW/1 -> Sum/5
  V_CEB/1 -> B5: V_CEB/1
  B5: V_CEB/1 -> Sum/6
  B6: Turbidity/1 -> Sum/7
  Feed Turbidity/1 -> B6: Turbidity/1
  T/1 -> B7: Temperature/1
  B7: Temperature/1 -> Sum/8

== system ARC_DTm/UF7/Subsystem ==
  note: The GAM utilizes smoothing functions to generate non-interacting linear regressions between the parameters. The format of the equation is as such:
      | $y = \beta_0 + \sum_{n=1}^N{f_n(x_n)}\\ f_n(x_n) = \beta_{n}*sm_n(x_n)$
      | where f_n is the weighted smoothing function for variable n across the set N. Each 1-D lookup table below represents the weighted smooth function output for the respective variable. This GAM lookup table approach provided a more computationally efficient method to predict using the GAM at very minor losses in fidelity ( ~0.1% MAPE from raw GAM outputs across a test set).
  t_BW : Inport
  t_CEB : Inport  Port=2
  t_CIP : Inport  Port=3
  V_BW : Inport  Port=4
  V_CEB : Inport  Port=5
  Feed Turbidity : Inport  Port=6
  T : Inport  Port=7
  B1: t_BW : Lookup_n-D  NumberOfTableDimensions=1  BreakpointsForDimension1=LUT.breakpoints(:,3)  Table=LUT.values(:,3)  ExtrapMethod=Clip  InternalRulePriority=Speed  RndMeth=Simplest
  B2: t_CEB : Lookup_n-D  NumberOfTableDimensions=1  BreakpointsForDimension1=LUT.breakpoints(:,5)  Table=LUT.values(:,5)  ExtrapMethod=Clip  InternalRulePriority=Speed  RndMeth=Simplest
  B3: t_CIP : Lookup_n-D  NumberOfTableDimensions=1  BreakpointsForDimension1=LUT.breakpoints(:,4)  Table=LUT.values(:,4)  ExtrapMethod=Clip  InternalRulePriority=Speed  RndMeth=Simplest
  B4: V_BW : Lookup_n-D  NumberOfTableDimensions=1  BreakpointsForDimension1=LUT.breakpoints(:,6)  Table=LUT.values(:,6)  ExtrapMethod=Clip  InternalRulePriority=Speed  RndMeth=Simplest
  B5: V_CEB : Lookup_n-D  NumberOfTableDimensions=1  BreakpointsForDimension1=LUT.breakpoints(:,7)  Table=LUT.values(:,7)  ExtrapMethod=Clip  InternalRulePriority=Speed  RndMeth=Simplest
  B6: Turbidity : Lookup_n-D  NumberOfTableDimensions=1  BreakpointsForDimension1=LUT.breakpoints(:,1)  Table=LUT.values(:,1)  ExtrapMethod=Clip  InternalRulePriority=Speed  RndMeth=Simplest
  B7: Temperature : Lookup_n-D  NumberOfTableDimensions=1  BreakpointsForDimension1=LUT.breakpoints(:,2)  Table=LUT.values(:,2)  ExtrapMethod=Clip  InternalRulePriority=Speed  RndMeth=Simplest
  Intercept : Constant  Value=LUT.intercept
  Sum : Sum  Inputs=++++++++
  A_UF : Outport
  wires:
  Sum/1 -> A_UF/1
  t_BW/1 -> B1: t_BW/1
  B1: t_BW/1 -> Sum/2
  Intercept/1 -> Sum/1
  t_CEB/1 -> B2: t_CEB/1
  B2: t_CEB/1 -> Sum/3
  t_CIP/1 -> B3: t_CIP/1
  B3: t_CIP/1 -> Sum/4
  V_BW/1 -> B4: V_BW/1
  B4: V_BW/1 -> Sum/5
  V_CEB/1 -> B5: V_CEB/1
  B5: V_CEB/1 -> Sum/6
  B6: Turbidity/1 -> Sum/7
  Feed Turbidity/1 -> B6: Turbidity/1
  T/1 -> B7: Temperature/1
  B7: Temperature/1 -> Sum/8

== system ARC_DTm/UF8/Subsystem ==
  note: The GAM utilizes smoothing functions to generate non-interacting linear regressions between the parameters. The format of the equation is as such:
      | $y = \beta_0 + \sum_{n=1}^N{f_n(x_n)}\\ f_n(x_n) = \beta_{n}*sm_n(x_n)$
      | where f_n is the weighted smoothing function for variable n across the set N. Each 1-D lookup table below represents the weighted smooth function output for the respective variable. This GAM lookup table approach provided a more computationally efficient method to predict using the GAM at very minor losses in fidelity ( ~0.1% MAPE from raw GAM outputs across a test set).
  t_BW : Inport
  t_CEB : Inport  Port=2
  t_CIP : Inport  Port=3
  V_BW : Inport  Port=4
  V_CEB : Inport  Port=5
  Feed Turbidity : Inport  Port=6
  T : Inport  Port=7
  B1: t_BW : Lookup_n-D  NumberOfTableDimensions=1  BreakpointsForDimension1=LUT.breakpoints(:,3)  Table=LUT.values(:,3)  ExtrapMethod=Clip  InternalRulePriority=Speed  RndMeth=Simplest
  B2: t_CEB : Lookup_n-D  NumberOfTableDimensions=1  BreakpointsForDimension1=LUT.breakpoints(:,5)  Table=LUT.values(:,5)  ExtrapMethod=Clip  InternalRulePriority=Speed  RndMeth=Simplest
  B3: t_CIP : Lookup_n-D  NumberOfTableDimensions=1  BreakpointsForDimension1=LUT.breakpoints(:,4)  Table=LUT.values(:,4)  ExtrapMethod=Clip  InternalRulePriority=Speed  RndMeth=Simplest
  B4: V_BW : Lookup_n-D  NumberOfTableDimensions=1  BreakpointsForDimension1=LUT.breakpoints(:,6)  Table=LUT.values(:,6)  ExtrapMethod=Clip  InternalRulePriority=Speed  RndMeth=Simplest
  B5: V_CEB : Lookup_n-D  NumberOfTableDimensions=1  BreakpointsForDimension1=LUT.breakpoints(:,7)  Table=LUT.values(:,7)  ExtrapMethod=Clip  InternalRulePriority=Speed  RndMeth=Simplest
  B6: Turbidity : Lookup_n-D  NumberOfTableDimensions=1  BreakpointsForDimension1=LUT.breakpoints(:,1)  Table=LUT.values(:,1)  ExtrapMethod=Clip  InternalRulePriority=Speed  RndMeth=Simplest
  B7: Temperature : Lookup_n-D  NumberOfTableDimensions=1  BreakpointsForDimension1=LUT.breakpoints(:,2)  Table=LUT.values(:,2)  ExtrapMethod=Clip  InternalRulePriority=Speed  RndMeth=Simplest
  Intercept : Constant  Value=LUT.intercept
  Sum : Sum  Inputs=++++++++
  A_UF : Outport
  wires:
  Sum/1 -> A_UF/1
  t_BW/1 -> B1: t_BW/1
  B1: t_BW/1 -> Sum/2
  Intercept/1 -> Sum/1
  t_CEB/1 -> B2: t_CEB/1
  B2: t_CEB/1 -> Sum/3
  t_CIP/1 -> B3: t_CIP/1
  B3: t_CIP/1 -> Sum/4
  V_BW/1 -> B4: V_BW/1
  B4: V_BW/1 -> Sum/5
  V_CEB/1 -> B5: V_CEB/1
  B5: V_CEB/1 -> Sum/6
  B6: Turbidity/1 -> Sum/7
  Feed Turbidity/1 -> B6: Turbidity/1
  T/1 -> B7: Temperature/1
  B7: Temperature/1 -> Sum/8

== system ARC_DTm/UF9/Subsystem ==
  note: The GAM utilizes smoothing functions to generate non-interacting linear regressions between the parameters. The format of the equation is as such:
      | $y = \beta_0 + \sum_{n=1}^N{f_n(x_n)}\\ f_n(x_n) = \beta_{n}*sm_n(x_n)$
      | where f_n is the weighted smoothing function for variable n across the set N. Each 1-D lookup table below represents the weighted smooth function output for the respective variable. This GAM lookup table approach provided a more computationally efficient method to predict using the GAM at very minor losses in fidelity ( ~0.1% MAPE from raw GAM outputs across a test set).
  t_BW : Inport
  t_CEB : Inport  Port=2
  t_CIP : Inport  Port=3
  V_BW : Inport  Port=4
  V_CEB : Inport  Port=5
  Feed Turbidity : Inport  Port=6
  T : Inport  Port=7
  B1: t_BW : Lookup_n-D  NumberOfTableDimensions=1  BreakpointsForDimension1=LUT.breakpoints(:,3)  Table=LUT.values(:,3)  ExtrapMethod=Clip  InternalRulePriority=Speed  RndMeth=Simplest
  B2: t_CEB : Lookup_n-D  NumberOfTableDimensions=1  BreakpointsForDimension1=LUT.breakpoints(:,5)  Table=LUT.values(:,5)  ExtrapMethod=Clip  InternalRulePriority=Speed  RndMeth=Simplest
  B3: t_CIP : Lookup_n-D  NumberOfTableDimensions=1  BreakpointsForDimension1=LUT.breakpoints(:,4)  Table=LUT.values(:,4)  ExtrapMethod=Clip  InternalRulePriority=Speed  RndMeth=Simplest
  B4: V_BW : Lookup_n-D  NumberOfTableDimensions=1  BreakpointsForDimension1=LUT.breakpoints(:,6)  Table=LUT.values(:,6)  ExtrapMethod=Clip  InternalRulePriority=Speed  RndMeth=Simplest
  B5: V_CEB : Lookup_n-D  NumberOfTableDimensions=1  BreakpointsForDimension1=LUT.breakpoints(:,7)  Table=LUT.values(:,7)  ExtrapMethod=Clip  InternalRulePriority=Speed  RndMeth=Simplest
  B6: Turbidity : Lookup_n-D  NumberOfTableDimensions=1  BreakpointsForDimension1=LUT.breakpoints(:,1)  Table=LUT.values(:,1)  ExtrapMethod=Clip  InternalRulePriority=Speed  RndMeth=Simplest
  B7: Temperature : Lookup_n-D  NumberOfTableDimensions=1  BreakpointsForDimension1=LUT.breakpoints(:,2)  Table=LUT.values(:,2)  ExtrapMethod=Clip  InternalRulePriority=Speed  RndMeth=Simplest
  Intercept : Constant  Value=LUT.intercept
  Sum : Sum  Inputs=++++++++
  A_UF : Outport
  wires:
  Sum/1 -> A_UF/1
  t_BW/1 -> B1: t_BW/1
  B1: t_BW/1 -> Sum/2
  Intercept/1 -> Sum/1
  t_CEB/1 -> B2: t_CEB/1
  B2: t_CEB/1 -> Sum/3
  t_CIP/1 -> B3: t_CIP/1
  B3: t_CIP/1 -> Sum/4
  V_BW/1 -> B4: V_BW/1
  B4: V_BW/1 -> Sum/5
  V_CEB/1 -> B5: V_CEB/1
  B5: V_CEB/1 -> Sum/6
  B6: Turbidity/1 -> Sum/7
  Feed Turbidity/1 -> B6: Turbidity/1
  T/1 -> B7: Temperature/1
  B7: Temperature/1 -> Sum/8

== system ARC_DTm/Plant_LocalLoad_FMU/Battery System/Basic Arbitrage ==
  Action Port : ActionPort  ActionPortLabel=elseif(u1==2)
  AND : Logic  IconShape=distinctive  AllPortsSameDT=off  OutDataTypeStr=Inherit: Inherit via back propagation
  AND1 : Logic  IconShape=distinctive  AllPortsSameDT=off  OutDataTypeStr=boolean
  Cast To Double : DataTypeConversion  OutDataTypeStr=double  SaturateOnIntegerOverflow=off  RndMeth=Floor
  Cast To Double1 : DataTypeConversion  OutDataTypeStr=double  SaturateOnIntegerOverflow=off  RndMeth=Floor
  Clock : Clock
  Minutes per day : Constant  Value=1440
  PeakDemandEnd : Constant  Value=21
  PeakDemandStart | SuperOffPeakEnd : Constant  Value=16
  Relational Operator : RelationalOperator  OutDataTypeStr=boolean  RndMeth=Simplest  InputSameDT=off
  Relational Operator1 : RelationalOperator  Operator=<=  OutDataTypeStr=boolean  RndMeth=Simplest  InputSameDT=off
  Relational Operator2 : RelationalOperator  OutDataTypeStr=boolean  RndMeth=Simplest  InputSameDT=off
  Relational Operator3 : RelationalOperator  Operator=<=  OutDataTypeStr=boolean  RndMeth=Simplest  InputSameDT=off
  Rem : Math  Operator=rem
  Scope : Scope  NumInputPorts=3
      settings: ActiveDisplayYMinimum=-2.9979166666666663  ActiveDisplayYMaximum=26.981250000000003  DataLoggingVariableName=ScopeData39
  SuperOffPeakStart : Constant  Value=11
  hour of day : Gain  Gain=1/60
  Battery Charge Command : Outport
  Battery Discharge Command : Outport  Port=2
  wires:
  Clock/1 -> Rem/1
  Minutes per day/1 -> Rem/2
  Rem/1 -> hour of day/1  "minute of day"
  hour of day/1 -> Relational Operator3/1, Relational Operator2/1, Relational Operator1/1, Scope/1, Relational Operator/1
  SuperOffPeakStart/1 -> Relational Operator/2
  Relational Operator/1 -> AND/1
  PeakDemandStart | SuperOffPeakEnd/1 -> Relational Operator2/2, Relational Operator1/2
  Relational Operator1/1 -> AND/2
  AND/1 -> Cast To Double/1  "SuperOffPeak"
  PeakDemandEnd/1 -> Relational Operator3/2
  Relational Operator2/1 -> AND1/1
  Relational Operator3/1 -> AND1/2
  AND1/1 -> Cast To Double1/1  "OnPeak"
  Cast To Double/1 -> Scope/2, Battery Charge Command/1
  Cast To Double1/1 -> Scope/3, Battery Discharge Command/1

== system ARC_DTm/Plant_LocalLoad_FMU/Battery System/Battery PID Solar Data ==
  note: M=2.5, kp=2.965, Ti=166.5, ki=0.0178
      |
      | M=1.5, kp=4.9, Ti=99.9, ki=0.049
      |
      | M=0.5, kp=14.8, Ti=33.3, ki=0.4
      |
      | M=0.1, kp=74.13, Ti=6.66, ki=11.13
      |
      | M=0.055 kp=134.79, Ti=3.663, ki=36.79
      |
      | M=0.01, kp=741.35, Ti=0.666, ki=1112.8
      |
      | M=0.001, kp=7413.5, Ti=0.0666, ki=111,313.81
      |
      | M=0.0001, kp=74135.09, Ti=0.00666, ki=11,113,394.89
  Setpoint : Inport
  feedback : Inport  Port=2
  Add : Sum
  BatteryCharge : Saturate  UpperLimit=1  LowerLimit=0
  Constant : Constant  Value=0
  Dead Zone : DeadZone  LowerValue=-0.01  UpperValue=0.01
  Dead Zone1 : DeadZone  LowerValue=-0.025  UpperValue=0.025
  Gain7 : Gain  Gain=134.79
  Gain8 : Gain  Gain=36.79
  Manual Switch : ManualSwitch
  Proportional3 : Gain  SaturateOnIntegerOverflow=on  OutDataTypeStr=Inherit: Same as input  ParamDataTypeStr=Inherit: Same as input
  Scope : Scope  NumInputPorts=3
      settings: ActiveDisplayYMinimum=-119.32425521603426  ActiveDisplayYMaximum=13.258250579559359  DataLoggingVariableName=ScopeData4
  Scope1 : Scope
      settings: ActiveDisplayYMinimum=-1  ActiveDisplayYMaximum=1  DataLoggingVariableName=ScopeData9
  Scope2 : Scope  NumInputPorts=4
      settings: Title=Setpoint  ActiveDisplayYMinimum=-0.96522618502196855  ActiveDisplayYMaximum=1.0322332055334107  DataLoggingVariableName=ScopeData2
  Scope3 : Scope  NumInputPorts=2
      settings: ActiveDisplayYMinimum=-0.25471317003362626  ActiveDisplayYMaximum=0.79251853030263664  DataLoggingVariableName=ScopeData2
  Subtract : Sum  Inputs=+-
  Subtract1 : Sum  Inputs=+-
  Sum1 : Sum  Inputs=|+-
  Sum6 : Sum  Inputs=+-  InputSameDT=on  SaturateOnIntegerOverflow=on  OutDataTypeStr=Inherit: Same as first input
  Unit Delay : UnitDelay  SampleTime=-1  HasFrameUpgradeWarning=on
  open-loop steps : Subsystem
  BatteryChargeDisch : Outport
  wires:
  Manual Switch/1 -> BatteryChargeDisch/1
  open-loop steps/1(Out1) -> Manual Switch/2
  Setpoint/1 -> Scope2/1, Subtract1/1
  Proportional3/1 -> Subtract/2
  feedback/1 -> Scope2/2, Subtract1/2
  Sum1/1 -> Add/2, Unit Delay/1
  Subtract/1 -> Scope1/1, Sum1/1
  Unit Delay/1 -> Sum1/2
  Subtract1/1 -> Scope3/2, Gain8/1, Gain7/1, Scope2/3, Scope3/1
  BatteryCharge/1 -> Scope2/4, Manual Switch/1, Sum6/2, Scope/2
  Add/1 -> Scope/1, Sum6/1, BatteryCharge/1
  Gain7/1 -> Add/1
  Gain8/1 -> Subtract/1
  Sum6/1 -> Proportional3/1, Scope/3
